simulink model "acrobot_sim_v1_PFL"  (R2013a)
settings: Solver=ode1  StartTime=0.0  StopTime=20  FixedStep=0.01  RelTol=1e-3
PreLoadFcn:
  | m1 = 1;
  | m2 = 1;
  | L1 = 1;
  | L2 = 1;
  | Lc1 = L1/2;
  | Lc2 = L2/2;
  | Ic1 = (Lc1*Lc1)/3;
  | Ic2 = (Lc2*Lc2)/3;
  | I1 = Ic1+m1*Lc1*Lc1;
  | I2 = Ic2+m2*Lc2*Lc2;
  | b1 = 0.4;
  | b2 = 0.4;
  | g = 9.8;
  | theta1_0 = -pi/8;
  | theta2_0 = -pi/3;
StartFcn:
  | m1 = 1;
  | m2 = 1;
  | L1 = 1;
  | L2 = 1;
  | Lc1 = L1/2;
  | Lc2 = L2/2;
  | Ic1 = (Lc1*Lc1)/3;
  | Ic2 = (Lc2*Lc2)/3;
  | I1 = Ic1+m1*Lc1*Lc1;
  | I2 = Ic2+m2*Lc2*Lc2;
  | b1 = 0.4;
  | b2 = 0.4;
  | g = 9.8;
  | theta1_0 = -pi/8;
  | theta2_0 = -pi/3;
libraries: mblibv1 x8, simulink x2
settings Model: Creator=Guy  LastModifiedBy=nightling
settings DataIOCC: SignalLoggingSaveFormat=ModelDataLogs
settings OptimizationCC: ExpressionDepthLimit=2147483647  InitFltsAndDblsToZero=on
settings DebuggingCC: FcnCallInpInsideContextMsg=UseLocalSettings  StrictBusMsg=Warning
settings SFSimCC: SimParseCustomCode=off
settings GRTTargetCC: CombineOutputUpdateFcns=off  GRTInterface=on
settings SimMechanicsCC: VisOnUpdateDiagram=on  VisDuringSimulation=on  AutoFitVis=GROWTOFIT  LastVizWinPosition=[685 679 560 420]  CamPosition=[0.997125;-1.39973;13.4628;]  CamTarget=[0.997125;-1.39973;0;]  CamUpVector=[0;1;0;]  CamHeight=3.22959  VisBackgroundColor=[0.9;0.9;0.95;]  DefaultBodyColor=[1;0;0;]

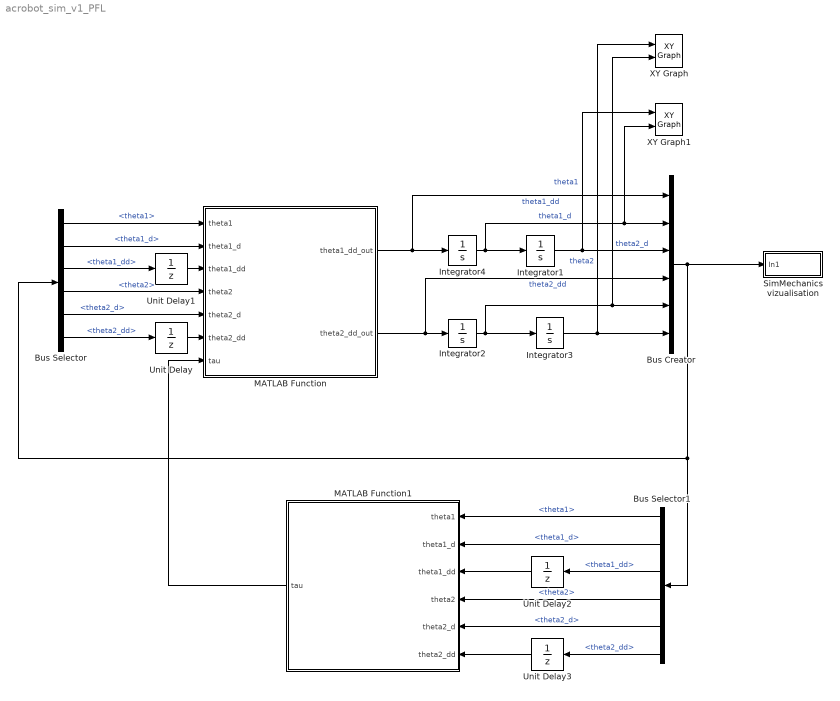
== system acrobot_sim_v1_PFL ==
  Bus Creator : BusCreator  Inputs=6
  Bus Selector : BusSelector  OutputSignals=theta1,theta1_d,theta1_dd,theta2,theta2_d,theta2_dd
  Bus Selector1 : BusSelector  OutputSignals=theta1,theta1_d,theta1_dd,theta2,theta2_d,theta2_dd
  Integrator1 : Integrator  InitialCondition=theta1_0
  Integrator2 : Integrator  InitialCondition="[0  ]"
  Integrator3 : Integrator  InitialCondition=theta2_0
  Integrator4 : Integrator  InitialCondition=[0 ]
  MATLAB Function : MATLAB Function
      settings: MinAlgLoopOccurrences=on
  MATLAB Function1 : MATLAB Function
      settings: MinAlgLoopOccurrences=on
  SimMechanics vizualisation : Subsystem
  Unit Delay{,1..3} (4 alike) : UnitDelay  SampleTime=-1
  XY Graph : simulink/Sinks/XY Graph  xmin=-0.5  xmax=0.5  ymin=-2  ymax=2  st=-1
  XY Graph1 : simulink/Sinks/XY Graph  xmin=-1  xmax=1  ymin=-5  ymax=5  st=-1
  wires:
  Integrator4/1 -> XY Graph1/2, Bus Creator/2, Integrator1/1  "theta1_d"
  Integrator1/1 -> XY Graph1/1, Bus Creator/3  "theta1"
  MATLAB Function/1(theta1_dd_out) -> Integrator4/1, Bus Creator/1  "theta1_dd"
  MATLAB Function/2(theta2_dd_out) -> Bus Creator/4, Integrator2/1  "theta2_dd"
  Integrator2/1 -> XY Graph/2, Bus Creator/5, Integrator3/1  "theta2_d"
  Integrator3/1 -> XY Graph/1, Bus Creator/6  "theta2"
  Bus Selector/1 -> MATLAB Function/1(theta1)  "<theta1>"
  Bus Selector/4 -> MATLAB Function/4(theta2)  "<theta2>"
  Bus Selector/6 -> Unit Delay/1  "<theta2_dd>"
  Bus Selector/5 -> MATLAB Function/5(theta2_d)  "<theta2_d>"
  Bus Selector/2 -> MATLAB Function/2(theta1_d)  "<theta1_d>"
  Bus Creator/1 -> Bus Selector1/1, Bus Selector/1, SimMechanics vizualisation/1(In1)
  Bus Selector/3 -> Unit Delay1/1  "<theta1_dd>"
  Unit Delay/1 -> MATLAB Function/6(theta2_dd)
  Unit Delay1/1 -> MATLAB Function/3(theta1_dd)
  Bus Selector1/1 -> MATLAB Function1/1(theta1)  "<theta1>"
  Bus Selector1/2 -> MATLAB Function1/2(theta1_d)  "<theta1_d>"
  Bus Selector1/3 -> Unit Delay2/1  "<theta1_dd>"
  Bus Selector1/4 -> MATLAB Function1/4(theta2)  "<theta2>"
  Bus Selector1/5 -> MATLAB Function1/5(theta2_d)  "<theta2_d>"
  Bus Selector1/6 -> Unit Delay3/1  "<theta2_dd>"
  MATLAB Function1/1(tau) -> MATLAB Function/7(tau)
  Unit Delay2/1 -> MATLAB Function1/3(theta1_dd)
  Unit Delay3/1 -> MATLAB Function1/6(theta2_dd)

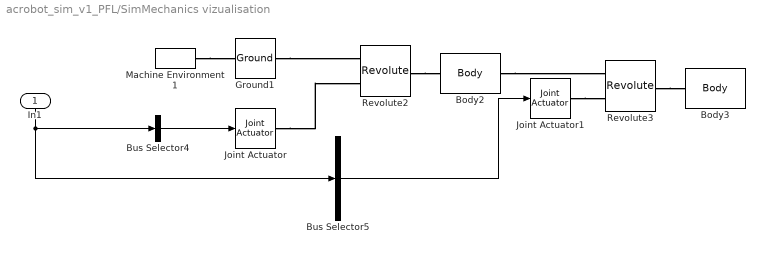
== system acrobot_sim_v1_PFL/SimMechanics vizualisation ==
  In1 : Inport
  Body2 : mblibv1/Bodies/Body  LConnTagsString=CS1  RConnTagsString=CS2  UpdateFromCAD=off  DialogClass=MechanicalBodyBlock  Mass=m1  MassUnits=kg  InertiaUnits=kg*m^2  Inertia=zeros(3)  Shape=Cylinder  ShapeDims=[1 1]  ShapeUnits=m  ShapeUse=false  Density=1  DensityUnits=kg/m^3  DensityUse=false  GraphicsMode=MACHINE_DEFAULT  BodyColorSelMode=COLORPALETTE  BodyColor=[0.043137 0.51765 0.78039]  AttachedToCS=CG  CG=Left$CG$[0 -L1/2 0]$CS1$CS1$m$[0 0 0]$Euler X-Y-Z$deg$WORLD$false$none  WorkingFrames=Left$CS1$[0 0 0]$Adjoining$Adjoining$m$[0 0 0]$Euler X-Y-Z$deg$WORLD$true$none#Right$CS2$[0 -L1 0]$CS1$CS1$m$[0 0 0]$Euler X-Y-Z$deg$WORLD$true$none  CGPos=[0 -L1/2 0]  CGRot=[0 0 0]  CS0Pos=[]  CS0Rot=[]  CS1Pos=[0 0 0]  CS1Rot=[0 0 0]  CS2Pos=[0 -L1 0]  CS2Rot=[0 0 0]  CS3Pos=[]  CS3Rot=[]  CS4Pos=[]  CS4Rot=[]  CS5Pos=[]  CS5Rot=[]  CS6Pos=[]  CS6Rot=[]  CS7Pos=[]  CS7Rot=[]  CS8Pos=[]  CS8Rot=[]  CS9Pos=[]  CS9Rot=[]  CS10Pos=[]  CS10Rot=[]  CS11Pos=[]  CS11Rot=[]  CS12Pos=[]  CS12Rot=[]  CS13Pos=[]  CS13Rot=[]  CS14Pos=[]  CS14Rot=[]  CS15Pos=[]  CS15Rot=[]  CS16Pos=[]  CS16Rot=[]  CS17Pos=[]  CS17Rot=[]  CS18Pos=[]  CS18Rot=[]  CS19Pos=[]  CS19Rot=[]  CS20Pos=[]  CS20Rot=[]
  Body3 : mblibv1/Bodies/Body  LConnTagsString=CS1  UpdateFromCAD=off  DialogClass=MechanicalBodyBlock  Mass=m2  MassUnits=kg  InertiaUnits=kg*m^2  Inertia=zeros(3)  Shape=Cylinder  ShapeDims=[1 1]  ShapeUnits=m  ShapeUse=false  Density=1  DensityUnits=kg/m^3  DensityUse=false  GraphicsMode=MACHINE_DEFAULT  BodyColorSelMode=COLORPALETTE  BodyColor=[0.043137 0.51765 0.78039]  AttachedToCS=CG  CG=Left$CG$[0 -L2/2 0]$CS1$CS1$m$[0 0 0]$Euler X-Y-Z$deg$WORLD$false$none  WorkingFrames=Left$CS1$[0 0 0]$Adjoining$Adjoining$m$[0 0 0]$Euler X-Y-Z$deg$WORLD$true$none#Right$CS2$[0 -L2 0]$CS1$CS1$m$[0 0 0]$Euler X-Y-Z$deg$WORLD$false$none  CGPos=[0 -L2/2 0]  CGRot=[0 0 0]  CS0Pos=[]  CS0Rot=[]  CS1Pos=[0 0 0]  CS1Rot=[0 0 0]  CS2Pos=[0 -L2 0]  CS2Rot=[0 0 0]  CS3Pos=[]  CS3Rot=[]  CS4Pos=[]  CS4Rot=[]  CS5Pos=[]  CS5Rot=[]  CS6Pos=[]  CS6Rot=[]  CS7Pos=[]  CS7Rot=[]  CS8Pos=[]  CS8Rot=[]  CS9Pos=[]  CS9Rot=[]  CS10Pos=[]  CS10Rot=[]  CS11Pos=[]  CS11Rot=[]  CS12Pos=[]  CS12Rot=[]  CS13Pos=[]  CS13Rot=[]  CS14Pos=[]  CS14Rot=[]  CS15Pos=[]  CS15Rot=[]  CS16Pos=[]  CS16Rot=[]  CS17Pos=[]  CS17Rot=[]  CS18Pos=[]  CS18Rot=[]  CS19Pos=[]  CS19Rot=[]  CS20Pos=[]  CS20Rot=[]
  Bus Selector4 : BusSelector  OutputSignals=theta1,theta1_d,theta1_dd  OutputAsBus=on
  Bus Selector5 : BusSelector  OutputSignals=theta2,theta2_d,theta2_dd  OutputAsBus=on
  Ground1 : mblibv1/Bodies/Ground  UpdateFromCAD=off  LeftPortType=env  RightPortType=workingframe  PhysicalDomain=Mechanical  DialogClass=GroundBlock  CoordPosition=[1 0 0]  CoordPositionUnits=m  StateVectorMgrId=0  MachineId=[1 0]  ShowEnvPort=on
  Joint Actuator : mblibv1/Sensors &  Actuators/Joint Actuator  UpdateFromCAD=off  PhysicalDomain=Mechanical  PortType=blob  ActuationStyle=Motion  AngleUnits=rad  ArcVelocityUnits=rad/s  ArcAccelerationUnits=rad/s^2  CoordPositionUnits=m  VelocityUnits=m/s  AccelerationUnits=m/s^2  ForceUnits=N  TorqueUnits=N*m  ActiveIO=on  Width=3  DialogClass=MechanicalActuatorBlock  Primitive=R1  ReferenceFrame=Absolute (World)
  Joint Actuator1 : mblibv1/Sensors &  Actuators/Joint Actuator  UpdateFromCAD=off  PhysicalDomain=Mechanical  PortType=blob  ActuationStyle=Motion  AngleUnits=rad  ArcVelocityUnits=rad/s  ArcAccelerationUnits=rad/s^2  CoordPositionUnits=m  VelocityUnits=m/s  AccelerationUnits=m/s^2  ForceUnits=N  TorqueUnits=N*m  ActiveIO=on  Width=3  DialogClass=MechanicalActuatorBlock  Primitive=R1  ReferenceFrame=Absolute (World)
  Machine Environment1 : mblibv1/Bodies/Machine Environment  PortType=env  PhysicalDomain=Mechanical  DialogTemplateClass=MECH.MachineEnvironment  SyncWhenCopied=off  Gravity=[0 -9.81 0]  GravityUnits=m/s^2  GravityAsSignal=off  Dimensionality=Auto-detect  AnalysisType=Forward dynamics  LinearAssemblyTolerance=1e-3  LinearAssemblyToleranceUnits=m  AngularAssemblyTolerance=1e-3  AngularAssemblyToleranceUnits=rad  ConstraintSolverType=Stabilizing  ConstraintRelTolerance=1e-4  ConstraintAbsTolerance=1e-4  UseRobustSingularityHandling=off  RedundancyAnalysisToleranceType=Automatically select tolerance  RedundancyAnalysisTolerance=1e-14  StatePerturbationType=Fixed  PerturbationSize=1e-5  VisualizeMachine=on  BodyVisualizationType=Use model default body geometries  BodyColorSelMode=Use model default  DefaultBodyColor=[1 0 0]
  Revolute2 : mblibv1/Joints/Revolute  LConnTagsString=__newl0|SA1  RConnTagsString=__newr0  UpdateFromCAD=off  NumSAPorts=1  CutJoint=off  MarkAsCut=off  Primitives=prismatic  PrimitiveProps=R1$World$[0 0 1]$revolute  DialogClass=JointBlock  R1Axis=[0 0 1]
  Revolute3 : mblibv1/Joints/Revolute  LConnTagsString=__newl0|SA1  RConnTagsString=__newr0  UpdateFromCAD=off  NumSAPorts=1  CutJoint=off  MarkAsCut=off  Primitives=prismatic  PrimitiveProps=R1$World$[0 0 1]$revolute  DialogClass=JointBlock  R1Axis=[0 0 1]
  wires:
  Bus Selector4/1 -> Joint Actuator/1
  In1/1 -> Bus Selector5/1, Bus Selector4/1
  Bus Selector5/1 -> Joint Actuator1/1
  connections:
  Revolute2/RConn1 -- Body2/LConn1
  Body2/RConn1 -- Revolute3/LConn1
  Revolute3/RConn1 -- Body3/LConn1
  Machine Environment1/RConn1 -- Ground1/LConn1
  Ground1/RConn1 -- Revolute2/LConn1
  Joint Actuator/RConn1 -- Revolute2/LConn2
  Joint Actuator1/RConn1 -- Revolute3/LConn2

== matlab function acrobot_sim_v1_PFL/MATLAB Function1 ==
  data: theta1 input; theta1_d input; theta1_dd input; theta2 input; theta2_d input; theta2_dd input; tau output; m1 parameter; m2 parameter; L1 parameter; L2 parameter; Lc1 parameter; Lc2 parameter; Ic1 parameter; Ic2 parameter; I1 parameter; I2 parameter; b1 parameter; b2 parameter; g parameter
function tau = PFL(theta1, theta1_d, theta1_dd, theta2, theta2_d, theta2_dd, m1, m2, L1, L2, Lc1, Lc2, Ic1, Ic2, I1, I2, b1, b2, g)
%#codegen
tau = I2*theta2_dd ...
      + (I2 + m2*L1*Lc2*cos(theta2))*theta1_dd ...
      + m2*L1*Lc2*sin(theta2)*theta1_d*theta1_d ...
      + b2*theta2_d ...
      + m2*g*Lc2*sin(theta1 + theta2) ...
      + 0;

== matlab function acrobot_sim_v1_PFL/MATLAB Function ==
  data: theta1 input; theta1_d input; theta1_dd input; theta1_dd_out output; theta2 input; theta2_d input; theta2_dd input; tau input; theta2_dd_out output; m1 parameter; m2 parameter; L1 parameter; L2 parameter; Lc1 parameter; Lc2 parameter; Ic1 parameter; Ic2 parameter; I1 parameter; I2 parameter; b1 parameter; b2 parameter; g parameter
function [theta1_dd_out, theta2_dd_out] = Acrobot(theta1, theta1_d, theta1_dd, theta2, theta2_d, theta2_dd, tau, m1, m2, L1, L2, Lc1, Lc2, Ic1, Ic2, I1, I2, b1, b2, g)
%#codegen
theta1_dd_out = (-(I2 + m2*L1*Lc2*cos(theta2))*theta2_dd ...
                + m2*L1*Lc2*sin(theta2)*(2*theta1_d*theta2_d + theta2_d*theta2_d) ...
                - b1*theta1_d ...
                - m1*g*Lc1*sin(theta1) ...
                - m2*g*(L1*sin(theta1) + Lc2*sin(theta1 + theta2))) ...
                / (I1 + I2 + m2*L1*(L1 + 2*Lc2*cos(theta2)));

theta2_dd_out = (-(I2 + m2*L1*Lc2*cos(theta2))*theta1_dd ...
                - m2*L1*Lc2*sin(theta2)*theta1_d*theta1_d ...
                - b2*theta2_d ...
                - m2*g*Lc2*sin(theta1 + theta2) ...
                + tau) ...
                / I2;
